simulink model "sim_PR_complete"  (R2015a)
settings: Solver=ode45  StartTime=0.0  StopTime=20  RelTol=1e-10  AbsTol=1e-10
values from neighbouring files (symbols this model uses):
  params = [g, m0, b0,                m1, I1, b1, L1, L1_cg,                m2, I2, b2, L2, L2_cg,                Kt, Ke, Ra, Vcc, D]    [load_params.m]    (also in load_single_params.m = [g, m0, b0,                m1, I1, b1, L1, L1_cg,           )
undefined symbols (not defined in the file or in its folder): m, n, p
settings Model: Creator=BPeixoto  LastModifiedBy=BPeixoto
settings SolverCC: AlgebraicLoopSolver=LineSearch
settings DataIOCC: LimitDataPoints=off
settings DebuggingCC: ArtificialAlgebraicLoopMsg=none

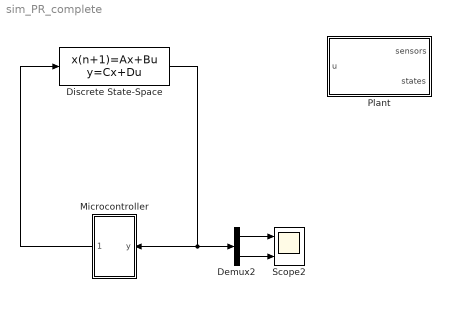
== system sim_PR_complete ==
  Demux2 : Demux  Outputs=2
  Discrete State-Space : DiscreteStateSpace  A=params.Phi  B=params.Gamma  C=params.C  D=params.D_  X0=[params.q0, params.qp0].'  SampleTime=params.ts
  Microcontroller : Subsystem
  Plant : Subsystem
  Scope2 : Scope  NumInputPorts=2
      settings: YMin=-5~-5  YMax=5~5
  wires:
  Microcontroller/1(PWM) -> Discrete State-Space/1
  Demux2/1 -> Scope2/1
  Demux2/2 -> Scope2/2
  Discrete State-Space/1 -> Microcontroller/1(y), Demux2/1

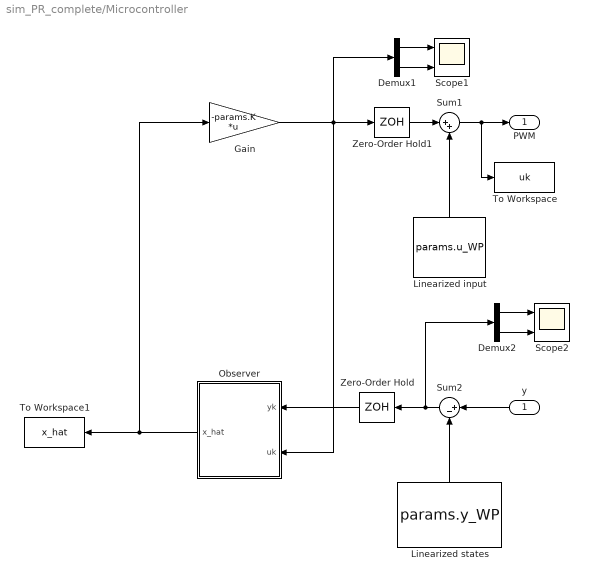
== system sim_PR_complete/Microcontroller ==
  y : Inport
  Demux1 : Demux  Outputs=2
  Demux2 : Demux  Outputs=2
  Gain : Gain  Gain=-params.K  Multiplication=Matrix(K*u) (u vector)
  Linearized input : Constant  Value=params.u_WP  VectorParams1D=off
  Linearized states : Constant  Value=params.y_WP  VectorParams1D=off
  Observer : Subsystem
  Scope1 : Scope  NumInputPorts=2
      settings: YMin=-1~-1.5  YMax=1.5~1  SaveName=ScopeData3
  Scope2 : Scope  NumInputPorts=2
      settings: YMin=-1~-1.5  YMax=1.5~1
  Sum1 : Sum  Inputs=|++
  Sum2 : Sum  Inputs=|+-
  To Workspace : ToWorkspace  VariableName=uk  SaveFormat=Structure With Time  SampleTime=-1
  To Workspace1 : ToWorkspace  VariableName=x_hat  SaveFormat=Structure With Time  SampleTime=-1
  Zero-Order Hold : ZeroOrderHold  SampleTime=params.ts
  Zero-Order Hold1 : ZeroOrderHold  SampleTime=params.ts
  PWM : Outport
  wires:
  Zero-Order Hold/1 -> Observer/1(yk)
  Zero-Order Hold1/1 -> Sum1/1
  Gain/1 -> Observer/2(uk), Demux1/1, Zero-Order Hold1/1
  Observer/1(x_hat) -> Gain/1, To Workspace1/1
  Linearized input/1 -> Sum1/2
  Demux1/1 -> Scope1/1
  Demux1/2 -> Scope1/2
  Sum1/1 -> To Workspace/1, PWM/1
  Linearized states/1 -> Sum2/2
  y/1 -> Sum2/1
  Sum2/1 -> Demux2/1, Zero-Order Hold/1
  Demux2/1 -> Scope2/1
  Demux2/2 -> Scope2/2

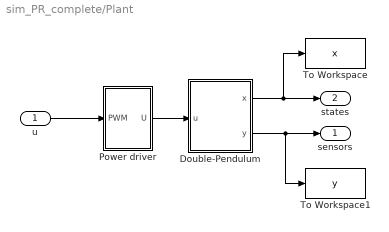
== system sim_PR_complete/Plant ==
  u : Inport
  Double-Pendulum : Subsystem
  Power driver : Subsystem
  To Workspace : ToWorkspace  VariableName=x  SaveFormat=Structure With Time  SampleTime=-1
  To Workspace1 : ToWorkspace  VariableName=y  SaveFormat=Structure With Time  SampleTime=-1
  sensors : Outport
  states : Outport  Port=2
  wires:
  Double-Pendulum/2(y) -> To Workspace1/1, sensors/1
  Double-Pendulum/1(x) -> states/1, To Workspace/1
  u/1 -> Power driver/1(PWM)
  Power driver/1(U) -> Double-Pendulum/1(u)

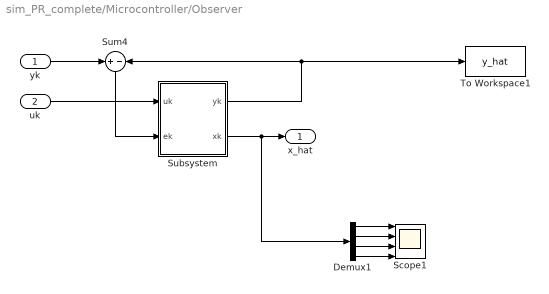
== system sim_PR_complete/Microcontroller/Observer ==
  yk : Inport
  uk : Inport  Port=2
  Demux1 : Demux
  Scope1 : Scope  NumInputPorts=4
      settings: YMin=-5~-5~-5~-5  YMax=5~5~5~5  SaveName=ScopeData5
  Subsystem : Subsystem
  Sum4 : Sum  Inputs=+|-
  To Workspace1 : ToWorkspace  VariableName=y_hat  SaveFormat=Structure With Time  SampleTime=-1
  x_hat : Outport
  wires:
  yk/1 -> Sum4/1
  Sum4/1 -> Subsystem/2(ek)
  Subsystem/1(yk) -> To Workspace1/1, Sum4/2
  uk/1 -> Subsystem/1(uk)
  Subsystem/2(xk) -> Demux1/1, x_hat/1
  Demux1/3 -> Scope1/3
  Demux1/4 -> Scope1/4
  Demux1/2 -> Scope1/2
  Demux1/1 -> Scope1/1

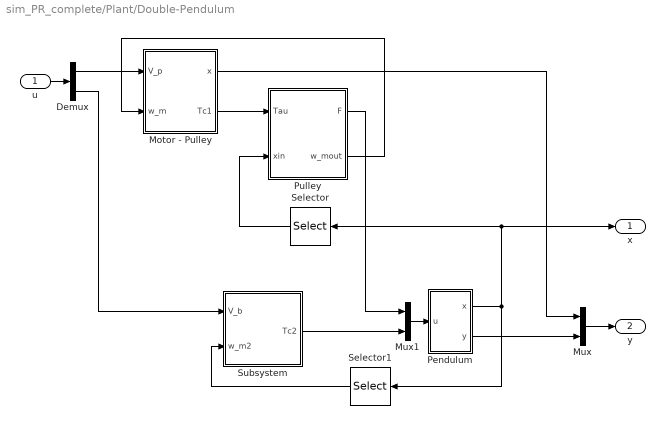
== system sim_PR_complete/Plant/Double-Pendulum ==
  u : Inport
  Demux : Demux  Outputs=2
  Motor - Pulley : Subsystem
  Mux : Mux  Inputs=2
  Mux1 : Mux  Inputs=2
  Pendulum : Subsystem
  Pulley : Subsystem
  Selector : Selector  InputPortWidth=4  Indices=[1]
  Selector1 : Selector  InputPortWidth=4  Indices=[4]
  Subsystem : Subsystem
  x : Outport
  y : Outport  Port=2
  wires:
  Pendulum/1(x) -> Selector1/1, x/1, Selector/1
  Mux/1 -> y/1
  Selector/1 -> Pulley/2(xin)
  Pendulum/2(y) -> Mux/2
  u/1 -> Demux/1
  Pulley/1(F) -> Mux1/1
  Mux1/1 -> Pendulum/1(u)
  Demux/1 -> Motor - Pulley/1(V_p)
  Pulley/2(w_mout) -> Motor - Pulley/2(w_m)
  Motor - Pulley/2(Tc1) -> Pulley/1(Tau)
  Motor - Pulley/1(x) -> Mux/1
  Demux/2 -> Subsystem/1(V_b)
  Selector1/1 -> Subsystem/2(w_m2)
  Subsystem/1(Tc2) -> Mux1/2

== system sim_PR_complete/Plant/Power driver ==
  PWM : Inport
  PWM-Tension conversion : Gain  Gain=params.Vcc  Multiplication=Matrix(K*u)
  U : Outport
  wires:
  PWM/1 -> PWM-Tension conversion/1
  PWM-Tension conversion/1 -> U/1

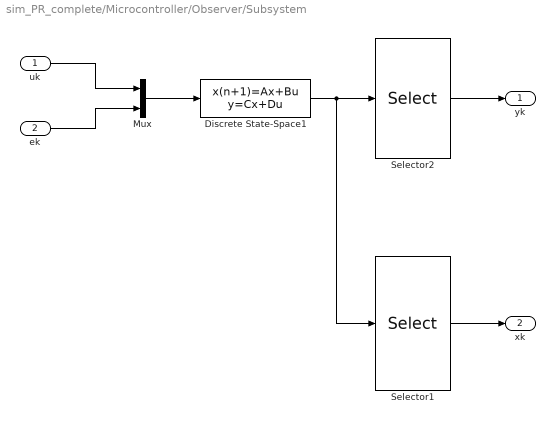
== system sim_PR_complete/Microcontroller/Observer/Subsystem ==
  uk : Inport
  ek : Inport  Port=2
  Discrete State-Space1 : DiscreteStateSpace  A=params.Phi  B=[params.Gamma, params.L]  C=[params.C; eye(length(params.x_WP))]  D=[params.D_, zeros(p, m); zeros(n, m), zeros(n, m)]  X0=zeros(size(params.x_WP))  SampleTime=params.ts
  Mux : Mux  Inputs=2
  Selector1 : Selector  InputPortWidth=6  Indices=[3 4 5 6]
  Selector2 : Selector  InputPortWidth=length(params.y_WP) + length(params.x_WP)  Indices=[1 2]
  yk : Outport
  xk : Outport  Port=2
  wires:
  Discrete State-Space1/1 -> Selector1/1, Selector2/1
  Mux/1 -> Discrete State-Space1/1
  uk/1 -> Mux/1
  ek/1 -> Mux/2
  Selector1/1 -> xk/1
  Selector2/1 -> yk/1

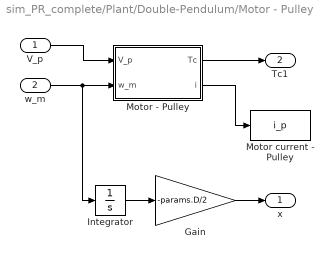
== system sim_PR_complete/Plant/Double-Pendulum/Motor - Pulley ==
  V_p : Inport
  w_m : Inport  Port=2
  Gain : Gain  Gain=-params.D/2
  Integrator : Integrator
  Motor - Pulley : MATLAB Function  TreatAsAtomicUnit=on
  Motor current - Pulley : ToWorkspace  VariableName=i_p  SaveFormat=Structure With Time  SampleTime=-1
  x : Outport
  Tc1 : Outport  Port=2
  wires:
  Motor - Pulley/2(i) -> Motor current - Pulley/1
  Motor - Pulley/1(Tc) -> Tc1/1
  w_m/1 -> Integrator/1, Motor - Pulley/2(w_m)
  Integrator/1 -> Gain/1
  Gain/1 -> x/1
  V_p/1 -> Motor - Pulley/1(V_p)

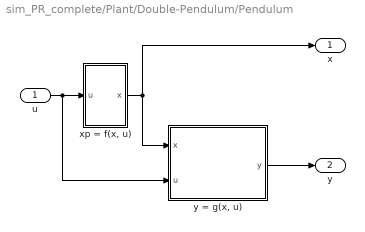
== system sim_PR_complete/Plant/Double-Pendulum/Pendulum ==
  u : Inport
  "xp = f(x, u)" : Subsystem
  "y = g(x, u)" : MATLAB Function  TreatAsAtomicUnit=on
  x : Outport
  y : Outport  Port=2
  wires:
  u/1 -> "y = g(x, u)"/2(u), "xp = f(x, u)"/1(u)
  "y = g(x, u)"/1(y) -> y/1
  "xp = f(x, u)"/1(x) -> x/1, "y = g(x, u)"/1(x)

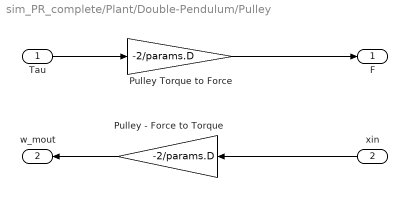
== system sim_PR_complete/Plant/Double-Pendulum/Pulley ==
  Tau : Inport
  xin : Inport  Port=2
  Pulley Torque to Force : Gain  Gain=-2/params.D
  Pulley - Force to Torque : Gain  Gain=-2/params.D
  F : Outport
  w_mout : Outport  Port=2
  wires:
  Pulley Torque to Force/1 -> F/1
  Tau/1 -> Pulley Torque to Force/1
  xin/1 -> Pulley - Force to Torque/1
  Pulley - Force to Torque/1 -> w_mout/1

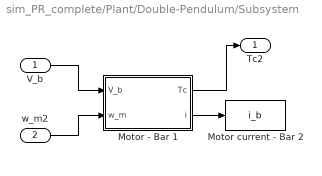
== system sim_PR_complete/Plant/Double-Pendulum/Subsystem ==
  V_b : Inport
  w_m2 : Inport  Port=2
  Motor - Bar 1 : MATLAB Function  TreatAsAtomicUnit=on
  Motor current - Bar 2 : ToWorkspace  VariableName=i_b  SaveFormat=Structure With Time  SampleTime=-1
  Tc2 : Outport
  wires:
  V_b/1 -> Motor - Bar 1/1(V_b)
  Motor - Bar 1/1(Tc) -> Tc2/1
  w_m2/1 -> Motor - Bar 1/2(w_m)
  Motor - Bar 1/2(i) -> Motor current - Bar 2/1

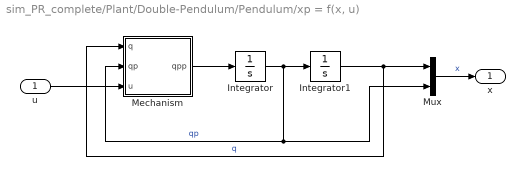
== system sim_PR_complete/Plant/Double-Pendulum/Pendulum/xp = f(x, u) ==
  u : Inport
  Integrator : Integrator  InitialCondition=params.qp0
  Integrator1 : Integrator  InitialCondition=params.q0
  Mechanism : Subsystem
  Mux : Mux  Inputs=2
  x : Outport
  wires:
  Mux/1 -> x/1  "x"
  u/1 -> Mechanism/3(u)
  Integrator/1 -> Integrator1/1, Mechanism/2(qp), Mux/2  "qp"
  Mechanism/1(qpp) -> Integrator/1
  Integrator1/1 -> Mux/1, Mechanism/1(q)  "q"

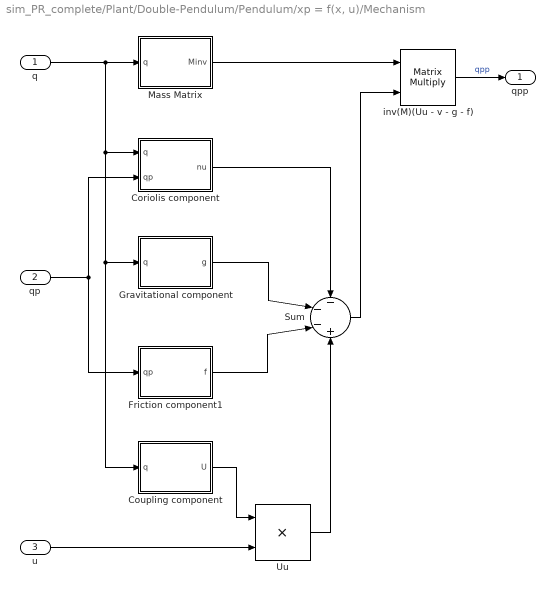
== system sim_PR_complete/Plant/Double-Pendulum/Pendulum/xp = f(x, u)/Mechanism ==
  q : Inport
  qp : Inport  Port=2
  u : Inport  Port=3
  Coriolis component : MATLAB Function  TreatAsAtomicUnit=on
  Coupling component : MATLAB Function  TreatAsAtomicUnit=on
  Friction component1 : MATLAB Function  TreatAsAtomicUnit=on
  Gravitational component : MATLAB Function  TreatAsAtomicUnit=on
  Mass Matrix : MATLAB Function  TreatAsAtomicUnit=on
  Sum : Sum  Inputs=-|-|-|+
  Uu : Product  RndMeth=Nearest
  inv(M)(Uu - v - g - f) : Product  Multiplication=Matrix(*)  OutDataTypeStr=Inherit: Inherit via back propagation  SaturateOnIntegerOverflow=on  InputSameDT=on
  qpp : Outport
  wires:
  Coriolis component/1(nu) -> Sum/1
  qp/1 -> Coriolis component/2(qp), Friction component1/1(qp)
  q/1 -> Coupling component/1(q), Gravitational component/1(q), Coriolis component/1(q), Mass Matrix/1(q)
  Gravitational component/1(g) -> Sum/2
  Friction component1/1(f) -> Sum/3
  Mass Matrix/1(Minv) -> inv(M)(Uu - v - g - f)/1
  Sum/1 -> inv(M)(Uu - v - g - f)/2
  inv(M)(Uu - v - g - f)/1 -> qpp/1  "qpp"
  Coupling component/1(U) -> Uu/1
  u/1 -> Uu/2
  Uu/1 -> Sum/4

== matlab function sim_PR_complete/Plant/Double-Pendulum/Pendulum/xp = f(x, u)/Mechanism/Coriolis component ==
  settings: updateMethod=DISCRETE  sampleTime=params.ts
  data: q input; qp input; nu output; params parameter
function nu = corvec(q, qp, params)
    nu = zeros(2, 1);

    % Coupled mass matrix
    nu(1) = -params.m1*params.L1_cg*(qp(2)^2)*sin(q(2));
    nu(2) = 0;
end

== matlab function sim_PR_complete/Plant/Double-Pendulum/Pendulum/xp = f(x, u)/Mechanism/Coupling component ==
  settings: updateMethod=DISCRETE  sampleTime=params.ts
  data: q input; U output
function U = Uvec(q)
    U = [1; 0];
end

== matlab function sim_PR_complete/Plant/Double-Pendulum/Subsystem/Motor - Bar 1 ==
  settings: updateMethod=DISCRETE  sampleTime=params.ts
  data: Tc output; i output; V_b input; w_m input; params parameter
function [Tc, i] = motor(V_b, w_m, params)
    % Motor parameters
    % Simplifications: 
    %   Negligible pulley inertia and stator inductance
    Ra = params.Ra;
    Kt = params.Kt;
    Ke = params.Ke;
    
    % Exerted Torque
    Tc = (Kt/Ra)*(V_b - Ke*w_m);
    i = Tc/Kt;
end

== matlab function sim_PR_complete/Plant/Double-Pendulum/Motor - Pulley/Motor - Pulley ==
  settings: updateMethod=DISCRETE  sampleTime=params.ts
  data: Tc output; i output; V_p input; w_m input; params parameter
function [Tc, i] = motor(V_p, w_m, params)
    % Motor parameters
    % Simplifications: 
    %   Negligible pulley inertia and stator inductance
    Ra = params.Ra;
    Kt = params.Kt;
    Ke = params.Ke;
    
    % Exerted Torque
    Tc = (Kt/Ra)*(V_p - Ke*w_m);
    i = Tc/Kt;
end

== matlab function sim_PR_complete/Plant/Double-Pendulum/Pendulum/xp = f(x, u)/Mechanism/Friction component1 ==
  settings: updateMethod=DISCRETE  sampleTime=params.ts
  data: qp input; f output; params parameter
function f = fvec(qp, params)
    f = zeros(2, 1);

    % Coupled mass matrix
    f(1) = params.b0*qp(1);
    f(2) = params.b1*qp(2);
end

== matlab function sim_PR_complete/Plant/Double-Pendulum/Pendulum/xp = f(x, u)/Mechanism/Gravitational component ==
  settings: updateMethod=DISCRETE  sampleTime=params.ts
  data: q input; g output; params parameter
function g = gvec(q, params)
    g = zeros(2, 1);

    % Coupled mass matrix
    g(1) = 0;
    g(2) = params.L1_cg*params.g*params.m1*sin(q(2));
end

== matlab function sim_PR_complete/Plant/Double-Pendulum/Pendulum/xp = f(x, u)/Mechanism/Mass Matrix ==
  settings: updateMethod=DISCRETE  sampleTime=params.ts
  data: q input; Minv output; params parameter
function Minv = mmatrix(q, params)
    M = zeros(2, 2);

    % Coupled mass matrix
    M(1,1) = params.m0 + params.m1;
    M(2,2) = params.m1*params.L1_cg^2 + params.I1;
    M(1,2) = params.m1*params.L1_cg*cos(q(2));
    M(1,2) = M(2,1);
    
    detM = M(1, 1)*M(2, 2) - M(1, 2)*M(2, 1);
    Minv = (1/detM)*[M(2, 2), -M(1, 2); -M(2, 1), M(1, 1)];
end

== matlab function sim_PR_complete/Plant/Double-Pendulum/Pendulum/y = g(x, u) ==
  settings: updateMethod=DISCRETE  sampleTime=params.ts
  data: x input; y output; u input
function y = system_output(x, u)
    y = x(2);
end
